simulink model "elevator_test"  (R2014a)
settings: Solver=ode45  StartTime=0.0  StopTime=1000000000.0  RelTol=1e-3
libraries: simulink x7
settings Model: Creator=Rishabh  LastModifiedBy=Rishabh

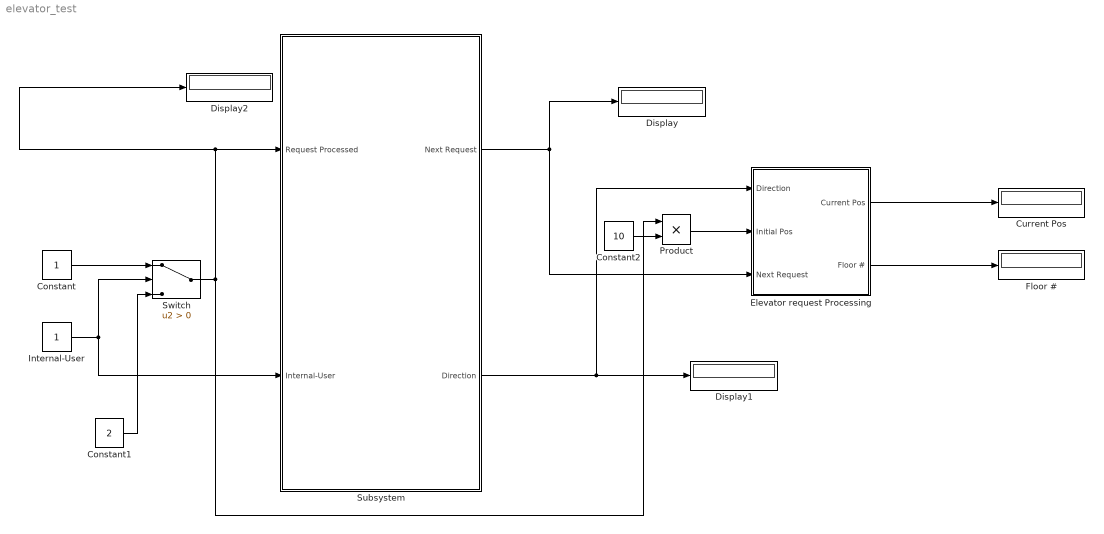
== system elevator_test ==
  Constant : Constant
  Constant1 : Constant  Value=2
  Constant2 : Constant  Value=10
  Current Pos : Display
  Display : Display
  Display1 : Display
  Display2 : Display
  Elevator request Processing : Subsystem
  Floor # : Display
  Internal-User : Constant
  Product : Product
  Subsystem : Subsystem
  Switch : Switch  Criteria=u2 > Threshold
  wires:
  Subsystem/2(Direction) -> Elevator request Processing/1(Direction), Display1/1
  Subsystem/1(Next Request) -> Display/1, Elevator request Processing/3(Next Request)
  Constant/1 -> Switch/1
  Internal-User/1 -> Subsystem/2(Internal-User), Switch/2
  Constant1/1 -> Switch/3
  Switch/1 -> Subsystem/1(Request Processed), Display2/1, Product/1
  Elevator request Processing/2(Floor #) -> Floor #/1
  Elevator request Processing/1(Current Pos) -> Current Pos/1
  Constant2/1 -> Product/2
  Product/1 -> Elevator request Processing/2(Initial Pos)

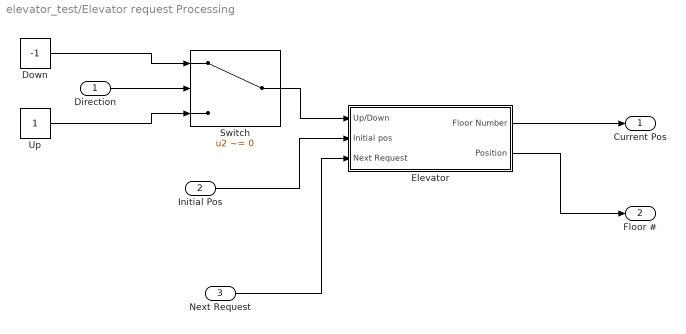
== system elevator_test/Elevator request Processing ==
  Direction : Inport
  Initial Pos : Inport  Port=2
  Next Request : Inport  Port=3
  Down : Constant  Value=-1
  Elevator : Subsystem
  Switch : Switch  Criteria=u2 ~= 0
  Up : Constant
  Current Pos : Outport
  Floor # : Outport  Port=2
  wires:
  Down/1 -> Switch/1
  Direction/1 -> Switch/2
  Switch/1 -> Elevator/1(Up/Down)
  Up/1 -> Switch/3
  Next Request/1 -> Elevator/3(Next Request)
  Elevator/1(Floor Number) -> Current Pos/1
  Elevator/2(Position) -> Floor #/1
  Initial Pos/1 -> Elevator/2(Initial pos)

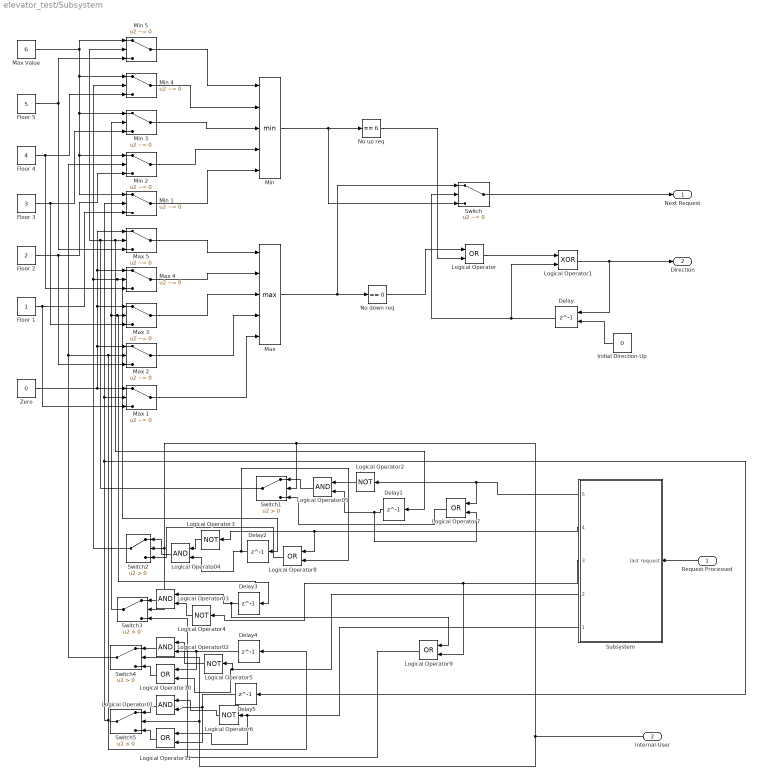
== system elevator_test/Subsystem ==
  Request Processed : Inport
  Internal-User : Inport  Port=2
  Delay : Delay  DelayLength=1  InitialConditionSource=Input port  InitialCondition=0  SampleTime=1
      settings: InputPortMap=u0,p4
  Delay{1..5} (5 alike) : Delay  DelayLength=1  InitialCondition=1  SampleTime=1
  Floor 1 : Constant
  Floor 2 : Constant  Value=2
  Floor 3 : Constant  Value=3
  Floor 4 : Constant  Value=4
  Floor 5 : Constant  Value=5
  Initial Direction-Up : Constant  Value=0  OutDataTypeStr=boolean
  Logical Operato04 : Logic  AllPortsSameDT=off  OutDataTypeStr=boolean
  Logical Operator{,7..11} (6 alike) : Logic  Operator=OR  AllPortsSameDT=off  OutDataTypeStr=boolean
  Logical Operator01 : Logic  AllPortsSameDT=off  OutDataTypeStr=boolean
  Logical Operator02 : Logic  AllPortsSameDT=off  OutDataTypeStr=boolean
  Logical Operator03 : Logic  AllPortsSameDT=off  OutDataTypeStr=boolean
  Logical Operator05 : Logic  AllPortsSameDT=off  OutDataTypeStr=boolean
  Logical Operator1 : Logic  Operator=XOR  AllPortsSameDT=off  OutDataTypeStr=boolean
  Logical Operator{2..6} (5 alike) : Logic  Operator=NOT  AllPortsSameDT=off  OutDataTypeStr=boolean
  Max : MinMax  Function=max  Inputs=5
  Max {1..5} (5 alike) : Switch  Criteria=u2 ~= 0
  Max Value : Constant  Value=6
  Min : MinMax  Inputs=5
  Min {1..4} (4 alike) : Switch  Criteria=u2 ~= 0
  Min 5 : Switch  Criteria=u2 ~= 0  Threshold=5
  No down req : simulink/Logic and Bit Operations/Compare To Constant  relop===  const=0  OutDataTypeStr=boolean
  No up req : simulink/Logic and Bit Operations/Compare To Constant  relop===  const=6  OutDataTypeStr=boolean
  Subsystem : Subsystem
  Switch : Switch  Criteria=u2 ~= 0
  Switch{1..5} (5 alike) : Switch  Criteria=u2 > Threshold
  Zero : Constant  Value=0
  Next Request : Outport
  Direction : Outport  Port=2
  wires:
  Initial Direction-Up/1 -> Delay/2
  Min 5/1 -> Min/1
  Floor 2/1 -> Max 2/3, Min 2/3
  Min 3/1 -> Min/3
  Logical Operator/1 -> Logical Operator1/1
  Delay/1 -> Switch/2, Logical Operator1/2
  Max 4/1 -> Max/2
  Min 1/1 -> Min/5
  Min 2/1 -> Min/4
  No down req/1 -> Logical Operator/1
  Logical Operator1/1 -> Direction/1, Delay/1
  Floor 1/1 -> Max 1/3, Min 1/3
  Min/1 -> Switch/3, No up req/1
  Floor 3/1 -> Max 3/3, Min 3/3
  Max Value/1 -> Min 5/1, Min 4/1, Min 3/1, Min 2/1, Min 1/1
  Floor 5/1 -> Min 5/3, Max 5/3
  Floor 4/1 -> Max 4/3, Min 4/3
  Max 5/1 -> Max/1
  Max 2/1 -> Max/4
  Switch/1 -> Next Request/1
  Max 1/1 -> Max/5
  Min 4/1 -> Min/2
  Zero/1 -> Max 5/1, Max 4/1, Max 3/1, Max 2/1, Max 1/1
  Max 3/1 -> Max/3
  No up req/1 -> Logical Operator/2
  Max/1 -> Switch/1, No down req/1
  Request Processed/1 -> Subsystem/1(last request)
  Switch1/1 -> Min 5/2, Delay1/1, Max 5/2
  Switch2/1 -> Min 4/2, Delay2/1, Max 4/2
  Switch3/1 -> Min 3/2, Delay3/1, Max 3/2
  Switch4/1 -> Min 2/2, Delay5/1, Min 1/2, Max 1/2, Delay4/1, Max 2/2
  Delay1/1 -> Logical Operator7/2, Logical Operator05/2
  Delay2/1 -> Logical Operator8/2, Logical Operato04/2
  Subsystem/2(4) -> Logical Operator8/1, Logical Operator3/1
  Subsystem/3(3) -> Logical Operator9/2, Logical Operator4/1
  Delay3/1 -> Logical Operator9/1, Logical Operator03/1
  Subsystem/4(2) -> Logical Operator10/2, Logical Operator5/1
  Delay4/1 -> Logical Operator10/1, Logical Operator02/2
  Delay5/1 -> Logical Operator11/2, Logical Operator01/2
  Subsystem/5(1) -> Logical Operator11/1, Logical Operator6/1
  Subsystem/1(5) -> Logical Operator7/1, Logical Operator2/1
  Logical Operator2/1 -> Logical Operator05/1
  Logical Operator3/1 -> Logical Operato04/1
  Logical Operator4/1 -> Logical Operator03/2
  Logical Operator5/1 -> Logical Operator02/1
  Logical Operator6/1 -> Logical Operator01/1
  Logical Operator7/1 -> Switch1/3
  Logical Operator05/1 -> Switch1/1
  Logical Operato04/1 -> Switch2/1
  Logical Operator8/1 -> Switch2/3
  Logical Operator9/1 -> Switch3/3
  Logical Operator03/1 -> Switch3/1
  Logical Operator02/1 -> Switch4/1
  Logical Operator10/1 -> Switch4/3
  Logical Operator01/1 -> Switch5/1
  Logical Operator11/1 -> Switch5/3
  Internal-User/1 -> Switch3/2, Switch2/2, Switch1/2, Switch4/2, Switch5/2

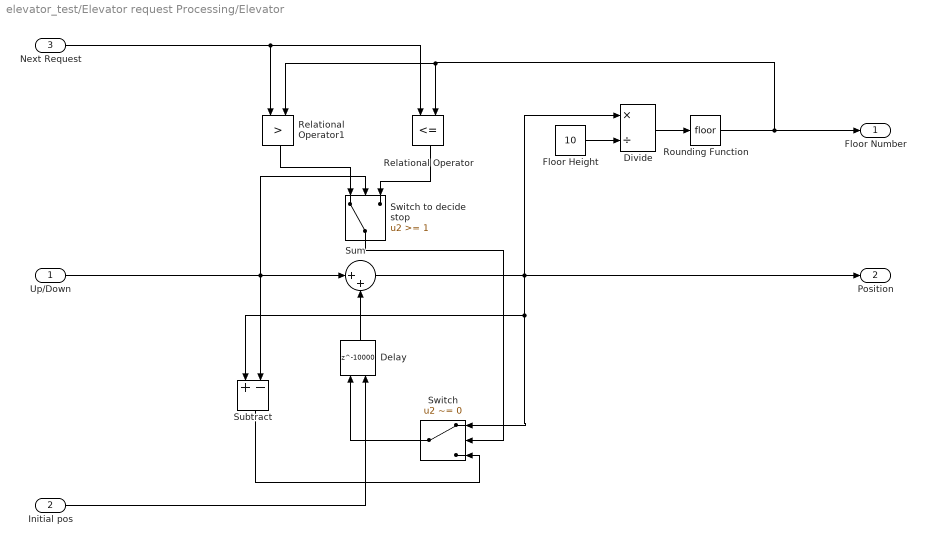
== system elevator_test/Elevator request Processing/Elevator ==
  Up/Down : Inport
  Initial pos : Inport  Port=2
  Next Request : Inport  Port=3
  Delay : Delay  DelayLength=10000  InitialConditionSource=Input port  InitialCondition=2  SampleTime=.00001
      settings: InputPortMap=u0,p4
  Divide : Product  Inputs=*/  RndMeth=Nearest  LockScale=on
  Floor Height : Constant  Value=10
  Relational Operator : RelationalOperator  Operator=<=  OutDataTypeStr=boolean
  Relational Operator1 : RelationalOperator  Operator=>  OutDataTypeStr=boolean
  Rounding Function : Rounding
  Subtract : Sum  Inputs=+-
  Sum : Sum  Inputs=|++
  Switch : Switch  Criteria=u2 ~= 0
  Switch to decide stop : Switch  Threshold=1
  Floor Number : Outport
  Position : Outport  Port=2
  wires:
  Delay/1 -> Sum/2
  Up/Down/1 -> Switch to decide stop/2, Sum/1, Subtract/2
  Sum/1 -> Position/1, Subtract/1, Switch/1, Divide/1
  Divide/1 -> Rounding Function/1
  Floor Height/1 -> Divide/2
  Rounding Function/1 -> Relational Operator1/2, Relational Operator/2, Floor Number/1
  Relational Operator/1 -> Switch to decide stop/3
  Next Request/1 -> Relational Operator1/1, Relational Operator/1
  Switch/1 -> Delay/1
  Relational Operator1/1 -> Switch to decide stop/1
  Switch to decide stop/1 -> Switch/2
  Subtract/1 -> Switch/3
  Initial pos/1 -> Delay/2

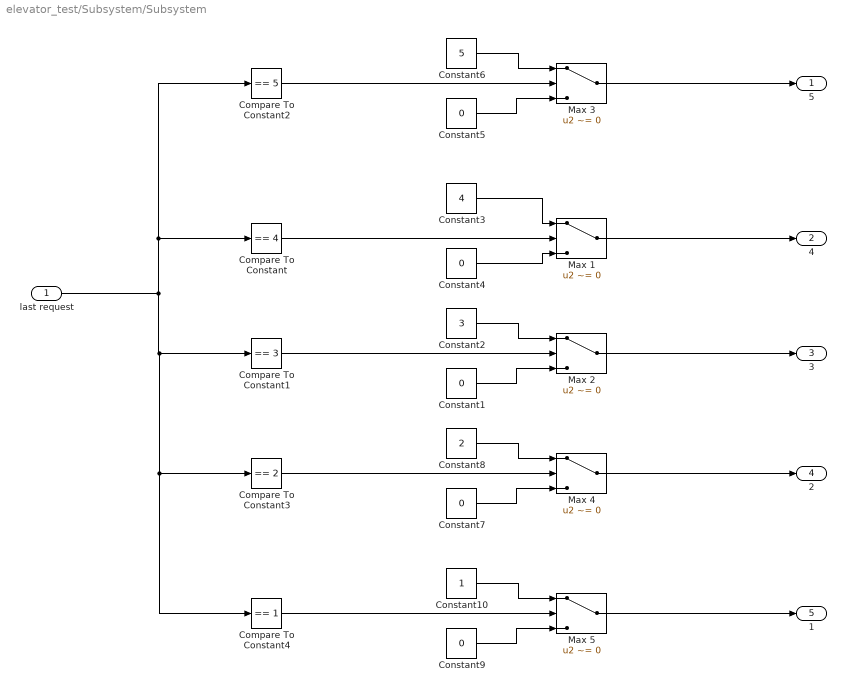
== system elevator_test/Subsystem/Subsystem ==
  last request : Inport
  Compare To Constant : simulink/Logic and Bit Operations/Compare To Constant  relop===  const=4  OutDataTypeStr=boolean
  Compare To Constant1 : simulink/Logic and Bit Operations/Compare To Constant  relop===  const=3  OutDataTypeStr=boolean
  Compare To Constant2 : simulink/Logic and Bit Operations/Compare To Constant  relop===  const=5  OutDataTypeStr=boolean
  Compare To Constant3 : simulink/Logic and Bit Operations/Compare To Constant  relop===  const=2  OutDataTypeStr=boolean
  Compare To Constant4 : simulink/Logic and Bit Operations/Compare To Constant  relop===  const=1  OutDataTypeStr=boolean
  Constant{1,4..5,7,9} (5 alike) : Constant  Value=0
  Constant10 : Constant
  Constant2 : Constant  Value=3
  Constant3 : Constant  Value=4
  Constant6 : Constant  Value=5
  Constant8 : Constant  Value=2
  Max {1..5} (5 alike) : Switch  Criteria=u2 ~= 0
  5 : Outport
  4 : Outport  Port=2
  3 : Outport  Port=3
  2 : Outport  Port=4
  1 : Outport  Port=5
  wires:
  Max 3/1 -> 5/1
  Constant5/1 -> Max 3/3
  Constant6/1 -> Max 3/1
  Compare To Constant2/1 -> Max 3/2
  Compare To Constant4/1 -> Max 5/2
  Max 5/1 -> 1/1
  Constant9/1 -> Max 5/3
  last request/1 -> Compare To Constant2/1, Compare To Constant/1, Compare To Constant4/1, Compare To Constant3/1, Compare To Constant1/1
  Constant10/1 -> Max 5/1
  Constant1/1 -> Max 2/3
  Max 1/1 -> 4/1
  Constant3/1 -> Max 1/1
  Compare To Constant1/1 -> Max 2/2
  Max 4/1 -> 2/1
  Constant7/1 -> Max 4/3
  Constant8/1 -> Max 4/1
  Compare To Constant3/1 -> Max 4/2
  Constant2/1 -> Max 2/1
  Compare To Constant/1 -> Max 1/2
  Max 2/1 -> 3/1
  Constant4/1 -> Max 1/3
